simulink model "Pacemaker_A2_06"  (R2020a)
settings: Solver=FixedStepAuto  StartTime=0.0  StopTime=10.0  FixedStep=1e-3  RelTol=1e-3  EnableMultiTasking=on
undefined symbols (not defined in the file): A0, A1, D0, D1, D10, D11, D12, D13, D2, D3, D4, D5, D6, D7, D8, D9, PTA0, PTA1, PTA2, PTB2, PTB23, PTB3, PTB9, PTC16, PTC17, PTC2, PTC3, PTC4, PTD0, PTD1, PTD2, PTD3
libraries: frdmk64flib x24, etargetslib x4
settings Model: ExtModeTrigDuration=5  Creator=forre  LastModifiedBy=forre
settings OptimizationCC: EnhancedBackFolding=on  PassReuseOutputArgsAs=Individual arguments  ZeroExternalMemoryAtStartup=off  ZeroInternalMemoryAtStartup=off  MaxStackSize=64  OptimizeBlockOrder=speed  DifferentSizesBufferReuse=on  OptimizationCustomize=off  EfficientTunableParamExpr=on
settings DebuggingCC: ParameterTunabilityLossMsg=error
settings HardwareCC: ProdBitPerPointer=32  ProdBitPerSizeT=32  ProdBitPerPtrDiffT=32  ProdLargestAtomicInteger=Long  ProdLargestAtomicFloat=Double  ProdWordSize=32  ProdHWDeviceType=ARM Compatible->ARM Cortex
settings SFSimCC: MATLABDynamicMemAlloc=off
settings RTWCC: SystemTargetFile=ert.tlc  HardwareBoard=NXP FRDM-K64F  TemplateMakefile=ert_default_tmf  Toolchain=GNU Tools for ARM Embedded Processors
settings CodeAppCC: ForceParamTrailComments=on  IgnoreCustomStorageClasses=off  OperatorAnnotations=on  SimulinkDataObjDesc=on  SFDataObjDesc=on  InsertBlockDesc=on

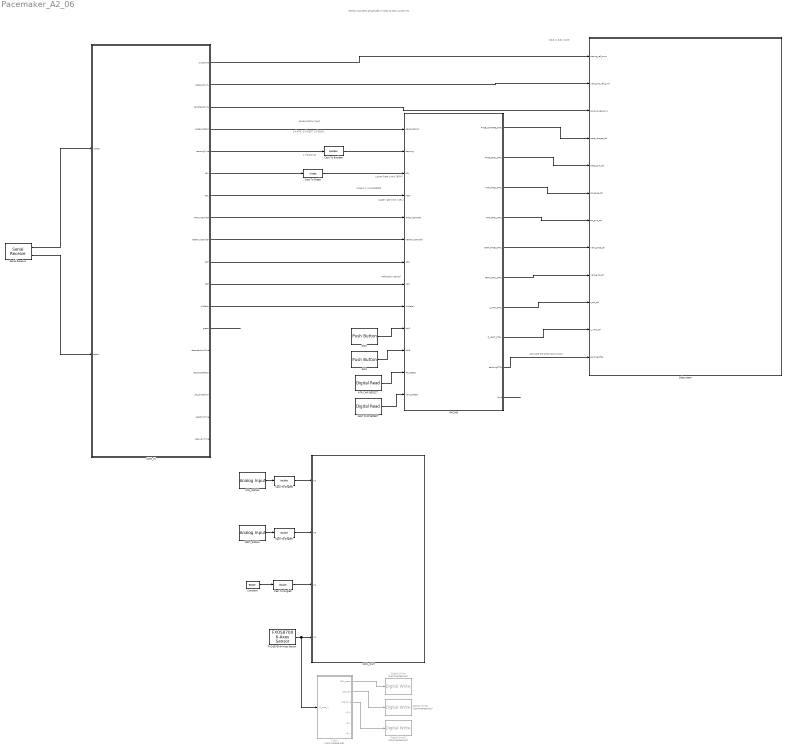
== system Pacemaker_A2_06 ==
  note: Python converts amplitude in Volts to duty cycle in %
  note: msecs = mins*60000
  note: Upper rate limit (URL)
  note: refractory period
  note: Lower Rate Limit (BPM)
  note: paceLocation input
  note: activate the sensing circuitry.
  note: 1 if ATR, 2 if VENT, 3 if DUAL
  note: input = duty cycle
  note: 1 if sensing
  ATR CMP DETECT : frdmk64flib/Digital Read  Whichpin=PTC16 (D0)  SampleTime=-1
  ATR_SIGNAL : frdmk64flib/Analog Input  Whichpin=PTB2 (A0)  SampleTime=-1
  COM_IN : Stateflow chart  TreatAsAtomicUnit=on
      settings: PortSchema="{\"entries\":[{\"content\":{\"sides\":[{\"content\":{\"connectorIds\":[\"In1\",\"In2\"]},\"type\":\"ConnectorPlacement.EquallySpacedRectSide\",\"uuid\":\"708f6c47-59ba-4c62-823e-aceb534f7d4e\"},{\"content\":{\"connectorIds\":[\"Out1\",\"Out3\",\"Out2\",\"Out4\",\"Out5\",\"Out6\",\"Out7\",\"Out8\",\"Out9\",\"Out10\",\"Out11\",\"Out12\",\"Out13\",\"Out14\",\"Out15\",\"Out16\",\"Out17\",\"Out18\"],\"side\":\"RIGHT\"},\"type\":\"ConnectorPlacement.EquallySpacedRectSide\",\"uuid\":\"fc195095-7643-467f-bfab-06db9c9b4f5e\"},{\"content\":{\"connectorIds\":[],\"side\":\"TOP\"},\"type\":\"ConnectorPlacement.EquallySpacedRectSide\",\"uuid\":\"2b9dc66d-b3fc-4626-8ab6-5dc1815dc2f6\"}]},\"type\":\"ConnectorPlacement.EquallySpacedConnector\",\"uuid\":\"ad24e883-72a0-4c10-9901-797c84f459ab\"}],\"packageUris\":[\"http://schema.mathworks.com/mf0/Connector/19700101\"],\"version\":\"1.0\"}"
  COM_OUT : Subsystem
  Cast To Boolean : DataTypeConversion  OutDataTypeStr=boolean
  Cast To Single : DataTypeConversion  OutDataTypeStr=single
  Cast To Single3 : DataTypeConversion  OutDataTypeStr=double
  Cast To Single5 : DataTypeConversion  OutDataTypeStr=double
  Cast To Single6 : DataTypeConversion  OutDataTypeStr=double
  Chart : Stateflow chart  Commented=on  TreatAsAtomicUnit=on
  Constant : Constant  Value=92020
  Digital Write : frdmk64flib/Digital Write  Commented=on  Whichpin=GREEN_LED
  Digital Write1 : frdmk64flib/Digital Write  Commented=on  Whichpin=RED_LED
  Digital Write7 : frdmk64flib/Digital Write  Commented=on  Whichpin=BLUE_LED
  FXOS8700 6-Axes Sensor : frdmk64flib/FXOS8700 6-Axes Sensor  Activesensor=Accelerometer only  ODR=800Hz  HybridODR=400Hz  Accelfullrange=-4g to +4g  SampleTime=-1
  PACING : Stateflow chart  TreatAsAtomicUnit=on
  SW2 : frdmk64flib/Push Button  Whichswitch=SW2  SampleTime1=-1
  SW3 : frdmk64flib/Push Button  Whichswitch=SW3  SampleTime1=-1
  Serial Receive : frdmk64flib/Serial Receive  SCIModule=0  Baudrate=uint32(9600)  Parity=None  StopBits=1  HardwareFlowControl=None  ByteOrder=LittleEndian  DataType=uint8  DataLength=38  BlockingMode=off  OutputStatus=on  SampleTime=-1
  Subsystem : Subsystem
  VENT CMP DETECT : frdmk64flib/Digital Read  Whichpin=PTC17 (D1)  SampleTime=-1
  VENT_SIGNAL : frdmk64flib/Analog Input  Whichpin=PTB3 (A1)  SampleTime=-1
  wires:
  SW2/1 -> PACING/10(btn2)
  PACING/4(ATR_GND_CTRL) -> Subsystem/7(atr_gnd_ctrl)
  PACING/3(ATR_PACE_CTRL) -> Subsystem/6(atr_pace_ctrl)
  PACING/1(PACE_CHARGE_CTRL) -> Subsystem/4(pace_charge_ctrl)
  PACING/2(PACE_GND_CTRL) -> Subsystem/5(pace_gnd_ctrl)
  PACING/5(VENT_PACE_CTRL) -> Subsystem/8(vent_pace_ctrl)
  PACING/6(VENT_GND_CTRL) -> Subsystem/9(vent_gnd_ctrl)
  PACING/7(Z_ATR_CTRL) -> Subsystem/10(z_atr_ctrl)
  PACING/8(Z_VENT_CTRL) -> Subsystem/11(" z_vent_ctrl")
  ATR CMP DETECT/1 -> PACING/12(atr_detect)
  VENT CMP DETECT/1 -> PACING/13(vent_detect)
  PACING/9(sensingCTRL) -> Subsystem/12(sensingCTRL)
  COM_IN/5(sensingTrue) -> Cast To Boolean/1
  PACING/10(blue) -> ?
  SW3/1 -> PACING/11(btn3)
  COM_IN/7(URL) -> PACING/4(MSR)
  COM_IN/10(ARP) -> PACING/7(ARP)
  COM_IN/11(VRP) -> PACING/8(VRP)
  Serial Receive/1 -> COM_IN/1(rxdata)
  Serial Receive/2 -> COM_IN/2(status)
  COM_IN/4(paceLocation) -> PACING/1(paceLocation)
  COM_IN/8(ATRpulseWidth) -> PACING/5(ATRpulseWidth)
  COM_IN/9(VENTpulseWidth) -> PACING/6(VENTpulseWidth)
  Cast To Boolean/1 -> PACING/2(sensing)
  COM_IN/6(LRL) -> Cast To Single/1
  Cast To Single/1 -> PACING/3(LRL)
  COM_IN/13(green) -> ?
  COM_IN/1(pulseAmp) -> Subsystem/1(pacing_ref_pwm)
  COM_IN/3(AtrSensitivity) -> Subsystem/2(vent_cmp_ref_pwm)
  COM_IN/2(VentSensitivity) -> Subsystem/3(atr_cmp_ref_pwm)
  COM_IN/12(AVdelay) -> PACING/9(AVdelay)
  Constant/1 -> Cast To Single3/1
  Cast To Single3/1 -> COM_OUT/3(In1)
  FXOS8700 6-Axes Sensor/1 -> Chart/1(AC_rate_in), COM_OUT/4(In4)
  VENT_SIGNAL/1 -> Cast To Single5/1
  ATR_SIGNAL/1 -> Cast To Single6/1
  Cast To Single5/1 -> COM_OUT/2(In3)
  Cast To Single6/1 -> COM_OUT/1(In2)
  Chart/1(LED_green) -> Digital Write/1
  Chart/2(LED_red) -> Digital Write1/1
  Chart/3(LED_blue) -> Digital Write7/1

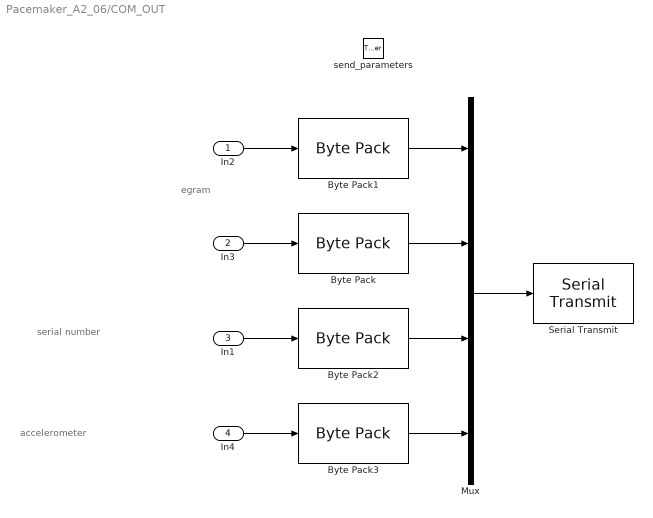
== system Pacemaker_A2_06/COM_OUT ==
  note: egram
  note: accelerometer
  note: serial number
  In2 : Inport
  In3 : Inport  Port=2
  In1 : Inport  Port=3
  In4 : Inport  Port=4
  send_parameters : TriggerPort  TriggerType=function-call  IsSimulinkFunction=on  FunctionName=send_parameters  VariantControl=(inherit)
  Byte Pack{,1..3} (4 alike) : etargetslib/Byte Pack  datatypes={'double'}  byteAlign=1
  Mux : Mux
  Serial Transmit : frdmk64flib/Serial Transmit  SCIModule=0  Baudrate=uint32(9600)  Parity=None  StopBits=1  HardwareFlowControl=None  ByteOrder=LittleEndian  BlockingMode=on  OutputStatus=off
  wires:
  Byte Pack/1 -> Mux/2
  Mux/1 -> Serial Transmit/1
  In3/1 -> Byte Pack/1
  In2/1 -> Byte Pack1/1
  Byte Pack1/1 -> Mux/1
  In1/1 -> Byte Pack2/1
  In4/1 -> Byte Pack3/1
  Byte Pack2/1 -> Mux/3
  Byte Pack3/1 -> Mux/4

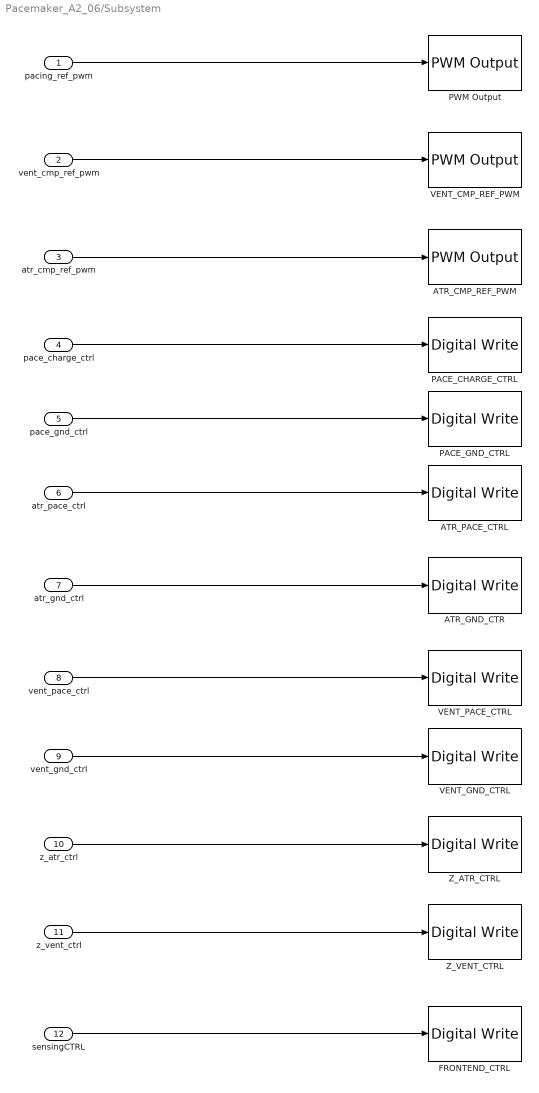
== system Pacemaker_A2_06/Subsystem ==
  pacing_ref_pwm : Inport
  vent_cmp_ref_pwm : Inport  Port=2
  atr_cmp_ref_pwm : Inport  Port=3
  pace_charge_ctrl : Inport  Port=4
  pace_gnd_ctrl : Inport  Port=5
  atr_pace_ctrl : Inport  Port=6
  atr_gnd_ctrl : Inport  Port=7
  vent_pace_ctrl : Inport  Port=8
  vent_gnd_ctrl : Inport  Port=9
  z_atr_ctrl : Inport  Port=10
  " z_vent_ctrl" : Inport  Port=11
  sensingCTRL : Inport  Port=12
  ATR_CMP_REF_PWM : frdmk64flib/PWM Output  Whichpin=PTC2 (D6)  InitialFrequency=2000  InitialDutyCycle=50
  ATR_GND_CTR : frdmk64flib/Digital Write  Whichpin=PTD2 (D11)
  ATR_PACE_CTRL : frdmk64flib/Digital Write  Whichpin=PTA0 (D8)
  FRONTEND_CTRL : frdmk64flib/Digital Write  Whichpin=PTD1 (D13)
  PACE_CHARGE_CTRL : frdmk64flib/Digital Write  Whichpin=PTB9 (D2)
  PACE_GND_CTRL : frdmk64flib/Digital Write  Whichpin=PTD0 (D10)
  PWM Output : frdmk64flib/PWM Output  Whichpin=PTA2 (D5)  InitialFrequency=2000  InitialDutyCycle=50
  VENT_CMP_REF_PWM : frdmk64flib/PWM Output  Whichpin=PTA1 (D3)  InitialFrequency=2000  InitialDutyCycle=50
  VENT_GND_CTRL : frdmk64flib/Digital Write  Whichpin=PTD3 (D12)
  VENT_PACE_CTRL : frdmk64flib/Digital Write  Whichpin=PTC4 (D9)
  Z_ATR_CTRL : frdmk64flib/Digital Write  Whichpin=PTB23 (D4)
  Z_VENT_CTRL : frdmk64flib/Digital Write  Whichpin=PTC3 (D7)
  wires:
  pace_gnd_ctrl/1 -> PACE_GND_CTRL/1
  atr_pace_ctrl/1 -> ATR_PACE_CTRL/1
  pace_charge_ctrl/1 -> PACE_CHARGE_CTRL/1
  atr_gnd_ctrl/1 -> ATR_GND_CTR/1
  vent_pace_ctrl/1 -> VENT_PACE_CTRL/1
  vent_gnd_ctrl/1 -> VENT_GND_CTRL/1
  z_atr_ctrl/1 -> Z_ATR_CTRL/1
  " z_vent_ctrl"/1 -> Z_VENT_CTRL/1
  sensingCTRL/1 -> FRONTEND_CTRL/1
  pacing_ref_pwm/1 -> PWM Output/1
  vent_cmp_ref_pwm/1 -> VENT_CMP_REF_PWM/1
  atr_cmp_ref_pwm/1 -> ATR_CMP_REF_PWM/1

== stateflow chart Pacemaker_A2_06/PACING ==
  note: beat sensed
  state SENSING_VENT_TRUE
    %sensing
  state VENT_CHARGING_AND_DISCHARGE
    entry:
    % for this state paceLocation = 1
    %begin charge and discharge cycle for ventricle
    msecPerPace = 60000.0/LRL; %new value in msec
    sensingCTRL = true; %enables the sensing circuitry if sensing = 1"
    ATR_PACE_CTRL = false;
    VENT_PACE_CTRL = false;
    PACE_CHARGE_CTRL = true;
    PACE_GND_CTRL = true;
    Z_VENT_CTRL = false;
    Z_ATR_CTRL = false
    VENT_GND_CTRL = true;
    ATR_GND_CTRL = false;
  state VENT_PACING
    entry:
    % pace ventricle
    PACE_GND_CTRL = true;
    VENT_PACE_CTRL = true;
    VENT_GND_CTRL = false;
    Z_VENT_CTRL = false;
    Z_ATR_CTRL = false;
    ATR_GND_CTRL = false;
    ATR_PACE_CTRL = false;
  note: VENT PACING
  note: switch to vent
  note: switch to atr
  state ATR_CHARGING_AND_DISCHARGE
    entry:
    % for this state paceLocation = 0
    %begin charge and discharge cycle for atrium
    msecPerPace = 60000.0/LRL; %new value for pace timing with msec units
    sensingCTRL = true; %enables the sensing circuitry if sensing = 1
    ATR_PACE_CTRL = false;
    VENT_PACE_CTRL = false;
    PACE_CHARGE_CTRL = true;
    PACE_GND_CTRL = true;
    Z_VENT_CTRL = false;
    Z_ATR_CTRL = false;
    VENT_GND_CTRL = false;
    ATR_GND_CTRL = true;
  state ATR_PACING
    entry:
    % pace atrium
    PACE_GND_CTRL = true;
    VENT_PACE_CTRL = false;
    VENT_GND_CTRL = false;
    Z_VENT_CTRL = false;
    Z_ATR_CTRL = false;
    ATR_GND_CTRL = false;
    ATR_PACE_CTRL = true;
  note: ATR PACING
  state SENSING_ATR_TRUE
    %sensing
  note: switch to atr
  note: beat sensed
  note: switch to dual
  state DUAL [commented out]
  VENT_PACING -> VENT_CHARGING_AND_DISCHARGE : after(VENTpulseWidth, msec)
  VENT_CHARGING_AND_DISCHARGE -> SENSING_VENT_TRUE [order 2] : after((VRP-VENTpulseWidth),msec)[sensing && (vent_detect || btn3)]
  SENSING_VENT_TRUE -> VENT_CHARGING_AND_DISCHARGE : after(VENTpulseWidth, msec)
  VENT_CHARGING_AND_DISCHARGE -> DUAL [commented out] : [paceLocation==3]
  DUAL -> VENT_CHARGING_AND_DISCHARGE [commented out]
  VENT_CHARGING_AND_DISCHARGE -> VENT_PACING [order 1] : after((msecPerPace-VENTpulseWidth), msec){PACE_CHARGE_CTRL = false;}
  ATR_CHARGING_AND_DISCHARGE -> VENT_CHARGING_AND_DISCHARGE [order 3] : [paceLocation==2]{blue=false;}
  VENT_CHARGING_AND_DISCHARGE -> ATR_CHARGING_AND_DISCHARGE [order 3] : [paceLocation==1]{blue=true;}
  (default) -> ATR_CHARGING_AND_DISCHARGE
  ATR_CHARGING_AND_DISCHARGE -> DUAL [commented out] : [paceLocation==3]
  ATR_CHARGING_AND_DISCHARGE -> ATR_PACING [order 1] : after((msecPerPace-ATRpulseWidth), msec){PACE_CHARGE_CTRL = false;}
  DUAL -> ATR_CHARGING_AND_DISCHARGE [commented out] : [paceLocation==1]
  ATR_PACING -> ATR_CHARGING_AND_DISCHARGE : after(ATRpulseWidth, msec)
  ATR_CHARGING_AND_DISCHARGE -> SENSING_ATR_TRUE [order 2] : after((ARP-ATRpulseWidth),msec)[sensing && (atr_detect || btn3)]
  SENSING_ATR_TRUE -> ATR_CHARGING_AND_DISCHARGE : after(ATRpulseWidth, msec)
  data: paceLocation input uint8; sensing input boolean; LRL input single; MSR input uint8; ATRpulseWidth input single; VENTpulseWidth input single; ARP input single; VRP input single; AVdelay input single; PACE_CHARGE_CTRL output boolean; PACE_GND_CTRL output boolean; btn2 input boolean; btn3 input boolean; ATR_PACE_CTRL output boolean; ATR_GND_CTRL output boolean; msecPerBeat local single; VENT_PACE_CTRL output boolean; VENT_GND_CTRL output boolean; Z_ATR_CTRL output boolean; Z_VENT_CTRL output boolean; atr_detect input boolean; vent_detect input boolean; sensingCTRL output boolean; msecPerPace local single; blue output boolean
  data paceLocation settings: description=|
      | 0 = pace atrium
      | 1 = pace ventricle
  data atr_detect settings: description=|
      | 0 = pace atrium
      | 1 = pace ventricle
  data vent_detect settings: description=|
      | 0 = pace atrium
      | 1 = pace ventricle

== stateflow chart Pacemaker_A2_06/Chart ==
  state LED_ON2
    entry:
    LED_red = true;
    LED_green = false;
  state LED_ON
    entry:
    LED_green = true;
    LED_red = false;
    LED_blue = false;
  state SET_AC
    entry:
    LED_green = false;
    LED_red = false;
    LED_blue = false;
  state Wait
    %wait
  state LED_ON3
    entry:
    LED_green = false;
    LED_green = false;
    LED_blue = true;
  LED_ON2 -> Wait
  Wait -> LED_ON2 [order 1] : after(1, sec)[AC_rate_in(1) > 0.1 || AC_rate_in(2) > 0.1 || AC_rate_in(3) > 0.1]
  (default) -> SET_AC
  Wait -> LED_ON [order 2] : after(1, sec)[AC_rate_in(1) > 0 && AC_rate_in(1) < 0.1]
  SET_AC -> Wait
  LED_ON -> Wait
  Wait -> LED_ON3 [order 3] : after(1, sec)[AC_rate_in(1) < 0]
  LED_ON3 -> Wait
  data: AC_rate_in input double; LED_green output boolean; LED_red output boolean; LED_blue output boolean; AC_z output; AC_y output; AC_x output

== stateflow chart Pacemaker_A2_06/COM_IN ==
  state SET_PARAMETERS
    entry:
    paceLocation = rxdata(3); %1 if ATRIUM, 2 if VENT, 3 if BOTH
    sensingTrue = rxdata(4); %1 if sensing, 0 if not
    LRL = rxdata(5);
    URL =  rxdata(6);
    AtrAmp = typecast(rxdata(7:10), 'single');
    VentAmp = typecast(rxdata(11:14),'single');
    ATRpulseWidth = typecast(rxdata(15:18),'single');
    VENTpulseWidth = typecast(rxdata(19:22),'single');
    ARP = typecast(rxdata(23:26),'single');
    VRP = typecast(rxdata(27:30),'single');
    AtrSensitivity = typecast(rxdata(31:34), 'single');
    VentSensitivity = typecast(rxdata(35:38), 'single');
    %AVdelay = typecast(rxdata(39:40), 'uint16');
    %rateAdaptive =  typecast(rxdata(31),'uint8');
  state INITIAL
    entry:
    paceLocation = 1; %1 if atr, 2 if vent, 3 if dual
    sensingTrue = 0; %1 if sensing, 0 if not
    LRL = 60; %ppm
    URL = 120; %ppm
    AtrAmp = 50; %duty cycle
    VentAmp = 50; %duty cycle
    ATRpulseWidth = 10; %msec
    VENTpulseWidth = 10; %msec
    ARP = 250; %msec
    VRP = 250; %msec
    AtrSensitivity = 50; %duty cycle
    VentSensitivity = 50; %duty cycle
    AVdelay = 50.0; %msec
    %other
    rateAdaptiveTrue = 0;
    acc_threshold = 20.5; %ajust according to Accelerometer single
    responseFactor = 1; % 1-16
    reactionTime = 10; % sec uint8
    recoveryTime = 30; % sec uint16
    %other
    green = false;
  note: receive values
  state STANDBY
    %waiting
  note: send values
  state ECHO_PARAMETERS
    entry:
    send_parameters();
  SET_PARAMETERS -> STANDBY [order 2] : [paceLocation==2]{pulseAmp = VentAmp;}
  SET_PARAMETERS -> STANDBY [order 1] : [paceLocation==1]{pulseAmp = AtrAmp;}
  (default) -> INITIAL
  (junction 14) -> SET_PARAMETERS [order 1] : [rxdata(2) == hex2dec('55')]
  (junction 18) -> STANDBY [order 2]
  INITIAL -> STANDBY
  STANDBY -> (junction 18) : [status==0]
  (junction 18) -> (junction 14) [order 1] : [rxdata(1) == hex2dec('16')]
  (junction 14) -> ECHO_PARAMETERS [order 2] : [rxdata(2) == hex2dec('22')]
  ECHO_PARAMETERS -> STANDBY
  data: pulseAmp output single; VentSensitivity output single; AtrSensitivity output single; paceLocation output uint8; sensingTrue output uint8; LRL output uint8; URL output uint8; ATRpulseWidth output single; VENTpulseWidth output single; ARP output single; rxdata input uint8; VRP output single; status input uint8; AtrAmp local single; VentAmp local single; AVdelay output single; green output boolean; rateAdaptiveTrue output uint8; responseFactor output uint8; acc_threshold output single; reactionTime output uint8; recoveryTime output uint8
